simulink model "pid_nn"  (R2023b)
settings: Solver=FixedStepAuto  StartTime=0.0  StopTime=20  FixedStep=1e-4  RelTol=1e-3
libraries: slpidlib x1
settings Model: Creator=Soumya Ranjan  LastModifiedBy=Soumya Ranjan

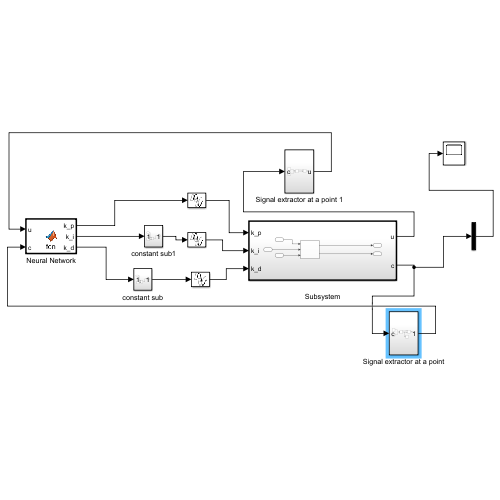
[thumbnail: Simulink's stored preview of the top-level diagram]
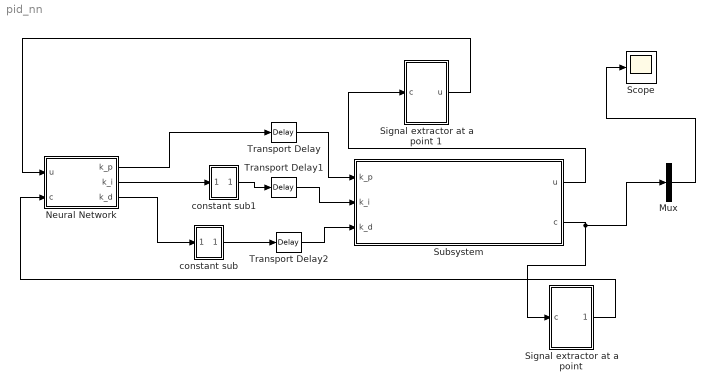
== system pid_nn ==
  " Subsystem" : Subsystem  TreatAsAtomicUnit=on
  Mux : Mux  Inputs=1
  Neural Network : MATLAB Function  TreatAsAtomicUnit=on
  Scope : Scope
  Signal extractor at a point : Subsystem
  Signal extractor at a point 1 : Subsystem
  Transport Delay : TransportDelay  DelayTime=0.1
  Transport Delay1 : TransportDelay  DelayTime=0.1
  Transport Delay2 : TransportDelay  DelayTime=0.1
  constant sub : Subsystem
  constant sub1 : Subsystem
  wires:
  " Subsystem"/2(c) -> Mux/1, Signal extractor at a point/1(c)
  Neural Network/1(k_p) -> Transport Delay/1
  Transport Delay/1 -> " Subsystem"/1(k_p)
  Transport Delay1/1 -> " Subsystem"/2(k_i)
  Transport Delay2/1 -> " Subsystem"/3(k_d)
  Signal extractor at a point/1(Out1) -> Neural Network/2(c)
  " Subsystem"/1(u) -> Signal extractor at a point 1/1(c)
  Signal extractor at a point 1/1(u) -> Neural Network/1(u)
  Mux/1 -> Scope/1
  Neural Network/3(k_d) -> constant sub/1(In1)
  constant sub/1(Out1) -> Transport Delay2/1
  Neural Network/2(k_i) -> constant sub1/1(In1)
  constant sub1/1(Out1) -> Transport Delay1/1

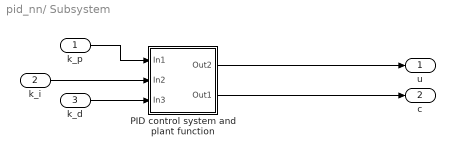
== system pid_nn/ Subsystem ==
  k_p : Inport
  k_i : Inport  Port=2
  k_d : Inport  Port=3
  PID control system and plant function : Subsystem
  u : Outport
  c : Outport  Port=2
  wires:
  PID control system and plant function/2(Out1) -> c/1
  PID control system and plant function/1(Out2) -> u/1
  k_p/1 -> PID control system and plant function/1(In1)
  k_i/1 -> PID control system and plant function/2(In2)
  k_d/1 -> PID control system and plant function/3(In3)

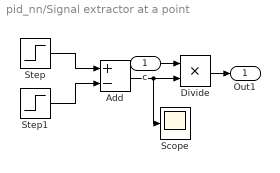
== system pid_nn/Signal extractor at a point ==
  c : Inport
  Add : Sum  Inputs=+-
  Divide : Product  Inputs=**
  Scope : Scope
  Step : Step  SampleTime=0
  Step1 : Step  Time=1.02  SampleTime=0
  Out1 : Outport
  wires:
  Step/1 -> Add/1
  Step1/1 -> Add/2
  c/1 -> Divide/1
  Add/1 -> Scope/1, Divide/2
  Divide/1 -> Out1/1

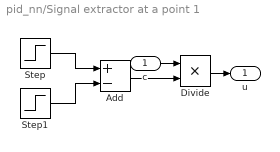
== system pid_nn/Signal extractor at a point 1 ==
  c : Inport
  Add : Sum  Inputs=+-
  Divide : Product  Inputs=**
  Step : Step  SampleTime=0
  Step1 : Step  Time=1.02  SampleTime=0
  u : Outport
  wires:
  Step/1 -> Add/1
  Step1/1 -> Add/2
  c/1 -> Divide/1
  Add/1 -> Divide/2
  Divide/1 -> u/1

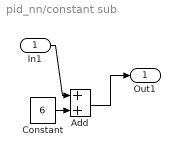
== system pid_nn/constant sub ==
  In1 : Inport
  Add : Sum
  Constant : Constant  Value=6
  Out1 : Outport
  wires:
  Add/1 -> Out1/1
  Constant/1 -> Add/2
  In1/1 -> Add/1

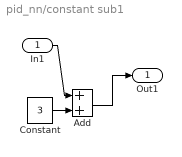
== system pid_nn/constant sub1 ==
  In1 : Inport
  Add : Sum
  Constant : Constant  Value=3
  Out1 : Outport
  wires:
  Add/1 -> Out1/1
  Constant/1 -> Add/2
  In1/1 -> Add/1

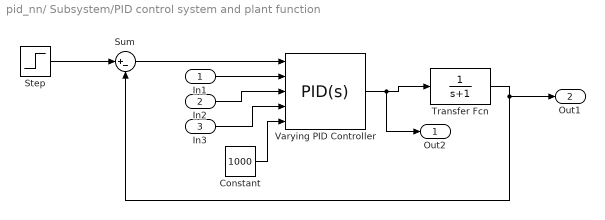
== system pid_nn/ Subsystem/PID control system and plant function ==
  In1 : Inport
  In2 : Inport  Port=2
  In3 : Inport  Port=3
  Constant : Constant  Value=1000
  Step : Step  Time=0  After=5  SampleTime=0
  Sum : Sum  Inputs=|+-
  Transfer Fcn : TransferFcn  Denominator=[1 1]
  Varying PID Controller : slpidlib/PID Controller  Controller=PID  Form=Parallel  TimeDomain=Continuous-time  UseExternalTs=off  SampleTime=0.1  IntegratorMethod=Forward Euler  FilterMethod=Forward Euler  ControllerParametersSource=external  P=1  I=1  UseKiTs=off  D=0  N=100  UseFilter=on  TunerSelectOption=Transfer Function Based (PID Tuner App)  InitialConditionSource=internal  InitialConditionForIntegrator=0  InitialConditionForFilter=0  DifferentiatorICPrevScaledInput=0  ExternalReset=none  TrackingMode=off  Kt=1  LimitOutput=off  SatLimitsSource=internal  UpperSaturationLimit=inf  LowerSaturationLimit=-inf  LinearizeAsGain=on  AntiWindupMode=none  Kb=1  LimitIntegrator=off  UpperIntegratorSaturationLimit=inf  LowerIntegratorSaturationLimit=-inf  POutMin=[]  POutMax=[]  IOutMin=[]  IOutMax=[]  DOutMin=[]  DOutMax=[]  NOutMin=[]  NOutMax=[]  SumOutMin=[]  SumOutMax=[]  SaturationOutMin=[]  SaturationOutMax=[]  PParamMin=[]  PParamMax=[]  IParamMin=[]  IParamMax=[]  DParamMin=[]  DParamMax=[]  NParamMin=[]  NParamMax=[]  KbParamMin=[]  KbParamMax=[]  KtParamMin=[]  KtParamMax=[]  KbOutMin=[]  KbOutMax=[]  KtOutMin=[]  KtOutMax=[]  IntegratorOutMin=[]  IntegratorOutMax=[]  FilterOutMin=[]  FilterOutMax=[]  SumI1OutMin=[]  SumI1OutMax=[]  SumI2OutMin=[]  SumI2OutMax=[]  SumI3OutMin=[]  SumI3OutMax=[]  SumI4OutMin=[]  SumI4OutMax=[]  SumDOutMin=[]  SumDOutMax=[]  DifferentiatorOutMin=[]  DifferentiatorOutMax=[]  FilterDiffOutCoefMin=[]  FilterDiffOutCoefMax=[]  ReciprocalOutMin=[]  ReciprocalOutMax=[]  SumDenOutMin=[]  SumDenOutMax=[]  SumNumOutMin=[]  SumNumOutMax=[]  DivideOutMin=[]  DivideOutMax=[]  UdiffTsProdOutMin=[]  UdiffTsProdOutMax=[]  NTsProdOutMin=[]  NTsProdOutMax=[]  UintegralTsProdOutMin=[]  UintegralTsProdOutMax=[]  UngainTsProdOutMin=[]  UngainTsProdOutMax=[]  ClampingZeroOutDataTypeStr=Inherit: Inherit via back propagation  ClampingZeroOutMin=[]  ClampingZeroOutMax=[]  FilterDenConstantOutDataTypeStr=Inherit: Inherit via back propagation  FilterDenConstantOutMin=[]  FilterDenConstantOutMax=[]  PCopyOutDataTypeStr=Inherit: Inherit via back propagation  PCopyOutMin=[]  PCopyOutMax=[]  NCopyOutDataTypeStr=Inherit: Inherit via back propagation  NCopyOutMin=[]  NCopyOutMax=[]  IntegratorContinuousStateAttributes=''  IntegratorStateMustResolveToSignalObject=off  IntegratorRTWStateStorageClass=Auto  FilterContinuousStateAttributes=''  FilterStateMustResolveToSignalObject=off  FilterRTWStateStorageClass=Auto  ParallelPVariant=ExternalParameters  IdealPVariant=Disabled  IVariant=ExternalParameters  DVariant=ExternalParameters  IntegratorVariant=Continuous  SatVariant=Disabled  AWVariant=Passthrough  PCopyVariant=Disabled  TRVariant=Disabled  FdbkBlocksVariant=Forward  IdealPFdbkVariant=Disabled  SatFdbkVariant=Disabled  DerivativeFilterVariant=ContFilter  NVariant=ExternalParameters  NCopyVariant=Disabled  FilterICVariant=InternalICsFilter  IntegratorICVariant=InternalICs  ExternalResetVariant=Disabled  TRSumVariant=Passthrough  SumFdbkVariant=Disabled  SumVariant=Sum_PID  TsampFilterVariant=InternalTs  TsampNgainVariant=Passthrough  TsampIntegralVariant=Disabled_SignalSpec  ExternalSaturationOutDataTypeStr=Inherit: Same as second input
      settings: LibrarySourceBlock=cstblocks/Linear Parameter Varying/Varying PID Controller
  Out2 : Outport
  Out1 : Outport  Port=2
  wires:
  Constant/1 -> Varying PID Controller/5
  Transfer Fcn/1 -> Out1/1, Sum/2
  In3/1 -> Varying PID Controller/4
  In1/1 -> Varying PID Controller/2
  Varying PID Controller/1 -> Out2/1, Transfer Fcn/1
  Sum/1 -> Varying PID Controller/1
  Step/1 -> Sum/1
  In2/1 -> Varying PID Controller/3

== matlab function pid_nn/Neural Network ==
  settings: updateMethod=DISCRETE
  data: u input; k_p output; c input; k_i output; k_d output
function [k_p,k_i,k_d] = fcn(u,c)
    [W_1,W_2,b]=layers(2,3,3);
    epoch=10;
  
    
    k_p=0;
    k_i= 0;
    k_d=0;


    delta_j=0.01;
    
    W_new_1=W_1;
    W_new_2=W_2;
    b_new=b;
    
    for i = 1:epoch
    
    
    
    
    
    
     
      
      X= [u;c];
    
      [O_j,O_k]=feedforward(X,W_1,W_2,b);
      k_p=O_k(1,1);
      k_i=O_k(2,1);
      k_d=O_k(3,1);
      [W_new_1,W_new_2,b_new,delta_j]=backpropagation(X,O_j,O_k,W_1,W_2,b,2,3,delta_j);
    
      
      
    end


function [weight_1,weight_2,bias] = layers(n_in,n_hidden,n_out)
    a = 0.5;
    b = 0.6;
    weight_1 = (b-a).*randn(n_hidden,n_in) + a;
    weight_2 = (b-a).*randn(n_out,n_hidden) + a;
    bias= (b-a).*randn(n_hidden,1) + a;
   




function [O_j,O_k] = feedforward(X,W_1,W_2,b)

  x_h= W_1*X +b;
  
  O_j = transpose(1/(1+exp(-x_h)));
  O_k= W_2*O_j;
  





function [W_1,W_2,b,s_delta_j]= backpropagation(X,O_j,O_k,W_1,W_2,b,alpha,beta,delta_j)
 
  delta_k=delta_j*sum(W_2)*O_k.*(1-O_k);
  
  slope_k= transpose(delta_k)*O_j ;

  delta_j= delta_k*sum(W_2)*O_j.*(1-O_j);
  slope_j= delta_j*(1/(1+exp(-X)));
  
  W_1 = W_1 + alpha*slope_j;
  W_2 = W_2 + alpha*slope_k;
  b = b - beta*delta_j;
  s_delta_j=sum(delta_j);
